simulink model "IS_2pulse_sim"  (R2025b)
settings: Solver=VariableStepAuto  StartTime=0.0  StopTime=10.0  RelTol=1e-3
values from neighbouring files (symbols this model uses):
  w_low = 2*pi*f_low    (= 314.159265359)    [IS_2pulse_main.m]
  w_res = f_res*2*pi    (= 1256.63706144)    [IS_2pulse_main.m]
  z_low = 0.7    [IS_2pulse_main.m]
  z_res = 0.02    [IS_2pulse_main.m]

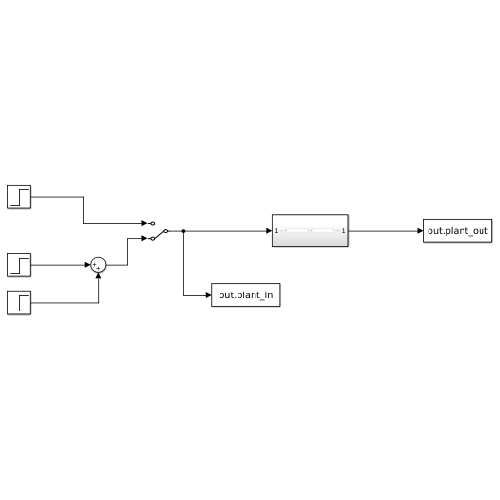
[thumbnail: Simulink's stored preview of the top-level diagram]
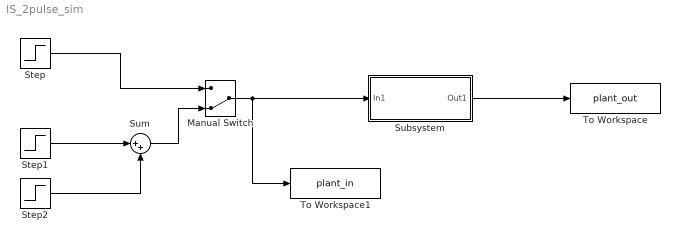
== system IS_2pulse_sim ==
  Manual Switch : ManualSwitch  CurrentSetting=0
  Step : Step  Time=0.05  SampleTime=0
  Step1 : Step  Time=0.05  After=0.5  SampleTime=0
  Step2 : Step  Time=0.0525  After=0.5  SampleTime=0
  Subsystem : Subsystem
  Sum : Sum  Inputs=|++
  To Workspace : ToWorkspace  VariableName=plant_out  SaveFormat=Timeseries  SampleTime=-1
  To Workspace1 : ToWorkspace  VariableName=plant_in  SaveFormat=Timeseries  SampleTime=-1
  wires:
  Manual Switch/1 -> To Workspace1/1, Subsystem/1(In1)
  Step/1 -> Manual Switch/1
  Sum/1 -> Manual Switch/2
  Step1/1 -> Sum/1
  Step2/1 -> Sum/2
  Subsystem/1(Out1) -> To Workspace/1

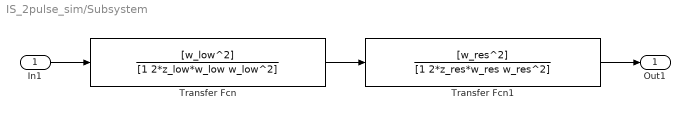
== system IS_2pulse_sim/Subsystem ==
  In1 : Inport
  Transfer Fcn : TransferFcn  Numerator=[w_low^2]  Denominator=[1 2*z_low*w_low w_low^2]
  Transfer Fcn1 : TransferFcn  Numerator=[w_res^2]  Denominator=[1 2*z_res*w_res w_res^2]
  Out1 : Outport
  wires:
  Transfer Fcn1/1 -> Out1/1
  Transfer Fcn/1 -> Transfer Fcn1/1
  In1/1 -> Transfer Fcn/1
